simulink model "tutorial43_advisor"  (R2025a)
settings: Solver=VariableStepAuto  StartTime=0.0  StopTime=10.0  RelTol=1e-3
settings Model: Creator=xing2  LastModifiedBy=xing2

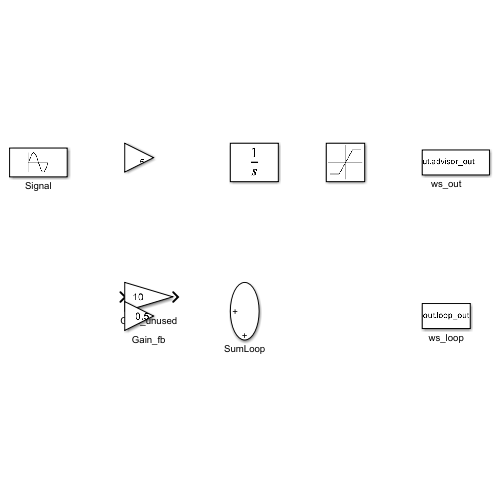
[thumbnail: Simulink's stored preview of the top-level diagram]
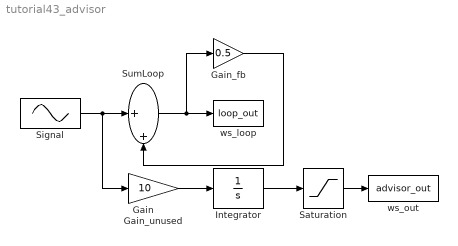
== system tutorial43_advisor ==
  Gain : Gain  Gain=5
  Gain_fb : Gain  Gain=0.5
  Gain_unused : Gain  Gain=10
  Integrator : Integrator
  Saturation : Saturate  UpperLimit=10  LowerLimit=-10
  Signal : Sin  SampleTime=0
  SumLoop : Sum  Inputs=|++
  ws_loop : ToWorkspace  VariableName=loop_out  SaveFormat=Timeseries  SampleTime=-1
  ws_out : ToWorkspace  VariableName=advisor_out  SaveFormat=Timeseries  SampleTime=-1
  wires:
  Signal/1 -> Gain/1, SumLoop/1
  Gain_fb/1 -> SumLoop/2
  SumLoop/1 -> Gain_fb/1, ws_loop/1
  Gain/1 -> Integrator/1
  Saturation/1 -> ws_out/1
  Integrator/1 -> Saturation/1
